simulink model "OREGO"  (Simulink 10.0)
settings: Solver=ode45  StartTime=0.0  StopTime=10.0  RelTol=1e-3  EnableMultiTasking=on
settings Model: Creator=tjohnson  LastModifiedBy=unknown
settings DataIOCC: LimitDataPoints=on
settings DebuggingCC: UnderspecifiedInitializationDetection=Simplified  MergeDetectMultiDrivingBlocksExec=error
settings GRTTargetCC: GeneratePreprocessorConditionals=Disable all  CombineOutputUpdateFcns=on  GRTInterface=off
settings ConfigComp: CovExternalEMLEnable=off

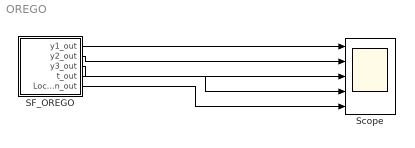
== system OREGO ==
  SF_OREGO : Stateflow chart  TreatAsAtomicUnit=on
  Scope : Scope  NumInputPorts=5
  wires:
  SF_OREGO/1(y1_out) -> Scope/1
  SF_OREGO/2(y2_out) -> Scope/2
  SF_OREGO/3(y3_out) -> Scope/3
  SF_OREGO/4(t_out) -> Scope/4
  SF_OREGO/5(Location_out) -> Scope/5

== stateflow chart SF_OREGO ==
  settings: updateMethod=CONTINUOUS
  state OREGO
    du:
    y1_dot = s * (y2 - y1 * y2 + y1 - q * y1 ^ 2.0);
    y2_dot = 1.0 / s * (-y2 - y1 * y2 + y3);
    y3_dot = w * (y1 - y3);
    t_dot = 1.0;
    y1_out=y1;
    y2_out=y2;
    y3_out=y3;
    t_out=t;
    Location_out =1;
  (default) -> OREGO : {t = 0.0; y1 = 1.0; y2 = 2.0; y3 = 3.0;}
  data: s constant double =77.27; q constant double =8.375e-06; w constant double =0.161; stop_time constant double =380; y1 local double; y1_out output double; y2 local double; y2_out output double; y3 local double; y3_out output double; t local double; t_out output double; Location_out output double
  data y1 settings: updateMethod=SF_CONTINUOUS_TIME_DATA
  data y2 settings: updateMethod=SF_CONTINUOUS_TIME_DATA
  data y3 settings: updateMethod=SF_CONTINUOUS_TIME_DATA
  data t settings: updateMethod=SF_CONTINUOUS_TIME_DATA
